simulink model "Simulink_Model_FL"  (R2022b)
settings: Solver=VariableStepAuto  StartTime=0.0  StopTime=10.0  RelTol=1e-3
settings Model: Creator=Owner  LastModifiedBy=Owner

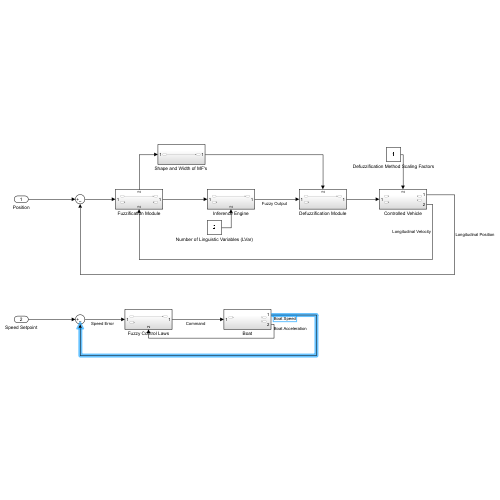
[thumbnail: Simulink's stored preview of the top-level diagram]
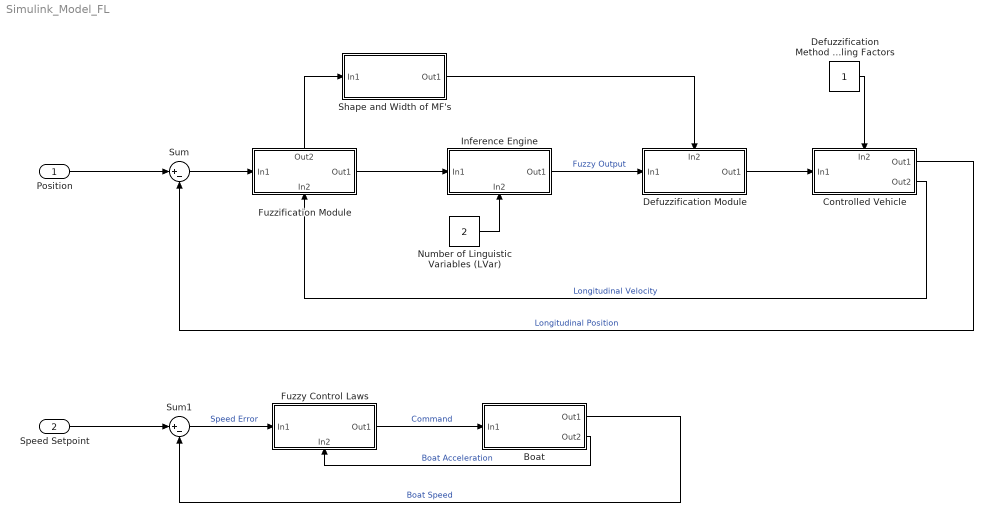
== system Simulink_Model_FL ==
  Position : Inport
  Speed Setpoint : Inport  Port=2
  Boat : Subsystem
  Controlled Vehicle : Subsystem
      settings: PortSchema="{\"entries\":[{\"content\":{\"sides\":[{\"content\":{\"connectorIds\":[\"In1\"]},\"type\":\"ConnectorPlacement.EquallySpacedRectSide\",\"uuid\":\"75031ec6-9104-4087-b797-3cb6d5dd7208\"},{\"content\":{\"connectorIds\":[\"Out1\",\"Out2\"],\"side\":\"RIGHT\"},\"type\":\"ConnectorPlacement.EquallySpacedRectSide\",\"uuid\":\"3dfb78db-9d63-4fd3-8e8c-d4df3b38d0df\"},{\"content\":{\"connectorIds\":[\"In2\"],\"side\":\"TOP\"},\"type\":\"ConnectorPlacement.EquallySpacedRectSide\",\"uuid\":\"5ad1c337-b1f5-4eed-a290-05ebccbcce06\"}]},\"type\":\"ConnectorPlacement.EquallySpacedConnector\",\"uuid\":\"4c9932b8-3cb4-4e36-bf01-1a56da01bb56\"}],\"packageUris\":[\"http://schema.mathworks.com/mf0/Connector/R2020b\"],\"version\":\"1.0\"}"
  Defuzzification Method Scaling Factors : Constant
  Defuzzification Module : Subsystem
      settings: PortSchema="{\"entries\":[{\"content\":{\"sides\":[{\"content\":{\"connectorIds\":[\"In1\"]},\"type\":\"ConnectorPlacement.EquallySpacedRectSide\",\"uuid\":\"328a4e44-e2ad-4c9f-8b0f-f73f2e04e1bb\"},{\"content\":{\"connectorIds\":[\"Out1\"],\"side\":\"RIGHT\"},\"type\":\"ConnectorPlacement.EquallySpacedRectSide\",\"uuid\":\"a69217c7-f31c-440f-b132-e8738ed85aa0\"},{\"content\":{\"connectorIds\":[\"In2\"],\"side\":\"TOP\"},\"type\":\"ConnectorPlacement.EquallySpacedRectSide\",\"uuid\":\"b5a7ef9f-e7ab-4f00-8acf-6718fb6dbd13\"}]},\"type\":\"ConnectorPlacement.EquallySpacedConnector\",\"uuid\":\"6d6e1eaf-78e5-45f3-b689-c36193959e3e\"}],\"packageUris\":[\"http://schema.mathworks.com/mf0/Connector/R2020b\"],\"version\":\"1.0\"}"
  Fuzzification Module : Subsystem
      settings: PortSchema="{\"entries\":[{\"content\":{\"sides\":[{\"content\":{\"connectorIds\":[\"In1\"]},\"type\":\"ConnectorPlacement.EquallySpacedRectSide\",\"uuid\":\"328a4e44-e2ad-4c9f-8b0f-f73f2e04e1bb\"},{\"content\":{\"connectorIds\":[\"Out1\"],\"side\":\"RIGHT\"},\"type\":\"ConnectorPlacement.EquallySpacedRectSide\",\"uuid\":\"a69217c7-f31c-440f-b132-e8738ed85aa0\"},{\"content\":{\"connectorIds\":[\"Out2\"],\"side\":\"TOP\"},\"type\":\"ConnectorPlacement.EquallySpacedRectSide\",\"uuid\":\"b5a7ef9f-e7ab-4f00-8acf-6718fb6dbd13\"},{\"content\":{\"connectorIds\":[\"In2\"],\"side\":\"BOTTOM\"},\"type\":\"ConnectorPlacement.EquallySpacedRectSide\",\"uuid\":\"f18c513e-db4e-4c5d-91df-32f50d8747fa\"}]},\"type\":\"ConnectorPlacement.EquallySpacedConnector\",\"uuid\":\"6d6e1eaf-78e5-45f3-b689-c36193959e3e\"}],\"packageUris\":[\"http://schema.mathworks.com/mf0/Connector/R2020b\"],\"version\":\"1.0\"}"
  Fuzzy Control Laws : Subsystem
      settings: PortSchema="{\"entries\":[{\"content\":{\"sides\":[{\"content\":{\"connectorIds\":[\"In1\"]},\"type\":\"ConnectorPlacement.EquallySpacedRectSide\",\"uuid\":\"328a4e44-e2ad-4c9f-8b0f-f73f2e04e1bb\"},{\"content\":{\"connectorIds\":[\"Out1\"],\"side\":\"RIGHT\"},\"type\":\"ConnectorPlacement.EquallySpacedRectSide\",\"uuid\":\"a69217c7-f31c-440f-b132-e8738ed85aa0\"},{\"content\":{\"connectorIds\":[],\"side\":\"TOP\"},\"type\":\"ConnectorPlacement.EquallySpacedRectSide\",\"uuid\":\"b5a7ef9f-e7ab-4f00-8acf-6718fb6dbd13\"},{\"content\":{\"connectorIds\":[\"In2\"],\"side\":\"BOTTOM\"},\"type\":\"ConnectorPlacement.EquallySpacedRectSide\",\"uuid\":\"f18c513e-db4e-4c5d-91df-32f50d8747fa\"}]},\"type\":\"ConnectorPlacement.EquallySpacedConnector\",\"uuid\":\"6d6e1eaf-78e5-45f3-b689-c36193959e3e\"}],\"packageUris\":[\"http://schema.mathworks.com/mf0/Connector/R2020b\"],\"version\":\"1.0\"}"
  Inference Engine : Subsystem
      settings: PortSchema="{\"entries\":[{\"content\":{\"sides\":[{\"content\":{\"connectorIds\":[\"In1\"]},\"type\":\"ConnectorPlacement.EquallySpacedRectSide\",\"uuid\":\"328a4e44-e2ad-4c9f-8b0f-f73f2e04e1bb\"},{\"content\":{\"connectorIds\":[\"Out1\"],\"side\":\"RIGHT\"},\"type\":\"ConnectorPlacement.EquallySpacedRectSide\",\"uuid\":\"a69217c7-f31c-440f-b132-e8738ed85aa0\"},{\"content\":{\"connectorIds\":[],\"side\":\"TOP\"},\"type\":\"ConnectorPlacement.EquallySpacedRectSide\",\"uuid\":\"b5a7ef9f-e7ab-4f00-8acf-6718fb6dbd13\"},{\"content\":{\"connectorIds\":[\"In2\"],\"side\":\"BOTTOM\"},\"type\":\"ConnectorPlacement.EquallySpacedRectSide\",\"uuid\":\"3f47bf65-3bf1-49d5-9f61-2c08bfefb51f\"}]},\"type\":\"ConnectorPlacement.EquallySpacedConnector\",\"uuid\":\"6d6e1eaf-78e5-45f3-b689-c36193959e3e\"}],\"packageUris\":[\"http://schema.mathworks.com/mf0/Connector/R2020b\"],\"version\":\"1.0\"}"
  Number of Linguistic Variables (LVar) : Constant  Value=2
  "Shape and Width of MF's " : Subsystem
  Sum : Sum  Inputs=|+-
  Sum1 : Sum  Inputs=|+-
  wires:
  Position/1 -> Sum/1
  Sum/1 -> Fuzzification Module/1(In1)
  Fuzzification Module/1(Out1) -> Inference Engine/1(In1)
  Inference Engine/1(Out1) -> Defuzzification Module/1(In1)  "Fuzzy Output"
  Defuzzification Module/1(Out1) -> Controlled Vehicle/1(In1)
  Controlled Vehicle/1(Out1) -> Sum/2  "Longitudinal Position"
  Controlled Vehicle/2(Out2) -> Fuzzification Module/2(In2)  "Longitudinal Velocity"
  Number of Linguistic Variables (LVar)/1 -> Inference Engine/2(In2)
  Fuzzification Module/2(Out2) -> "Shape and Width of MF's "/1(In1)
  "Shape and Width of MF's "/1(Out1) -> Defuzzification Module/2(In2)
  Defuzzification Method Scaling Factors/1 -> Controlled Vehicle/2(In2)
  Speed Setpoint/1 -> Sum1/1
  Sum1/1 -> Fuzzy Control Laws/1(In1)  "Speed Error"
  Fuzzy Control Laws/1(Out1) -> Boat/1(In1)  "Command"
  Boat/1(Out1) -> Sum1/2  "Boat Speed"
  Boat/2(Out2) -> Fuzzy Control Laws/2(In2)  "Boat Acceleration"

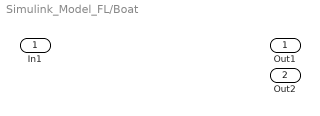
== system Simulink_Model_FL/Boat ==
  In1 : Inport
  Out1 : Outport
  Out2 : Outport  Port=2

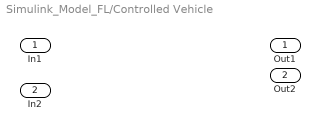
== system Simulink_Model_FL/Controlled Vehicle ==
  In1 : Inport
  In2 : Inport  Port=2
  Out1 : Outport
  Out2 : Outport  Port=2

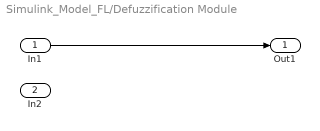
== system Simulink_Model_FL/Defuzzification Module ==
  In1 : Inport
  In2 : Inport  Port=2
  Out1 : Outport
  wires:
  In1/1 -> Out1/1

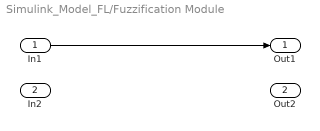
== system Simulink_Model_FL/Fuzzification Module ==
  In1 : Inport
  In2 : Inport  Port=2
  Out1 : Outport
  Out2 : Outport  Port=2
  wires:
  In1/1 -> Out1/1

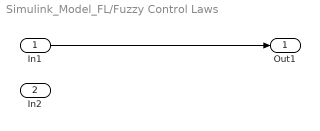
== system Simulink_Model_FL/Fuzzy Control Laws ==
  In1 : Inport
  In2 : Inport  Port=2
  Out1 : Outport
  wires:
  In1/1 -> Out1/1

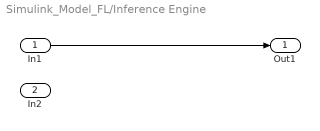
== system Simulink_Model_FL/Inference Engine ==
  In1 : Inport
  In2 : Inport  Port=2
  Out1 : Outport
  wires:
  In1/1 -> Out1/1

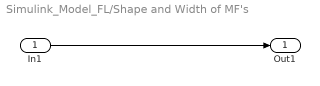
== system Simulink_Model_FL/Shape and Width of MF's  ==
  In1 : Inport
  Out1 : Outport
  wires:
  In1/1 -> Out1/1
